simulink model "untitled"  (R2021a)
settings: Solver=VariableStepAuto  StartTime=0.0  StopTime=10  RelTol=1e-3
undefined symbols (not defined in the file or in its folder): magnitude, X, Y, Z
libraries: nesl_utility x14, sm_lib x7, aerolibnav x4, ee_lib x1
settings Model: Creator=thana  LastModifiedBy=thana
settings ExplorerConfigSet: InternalSimMechanicsExplorerSettings="<ExplorerConfiguration><canonicalview>planar_xy</canonicalview><AnimationSetting><BasePlaybackSpeed>1.0</BasePlaybackSpeed><PlaybackSpeedFactor>0.00390625</PlaybackSpeedFactor></AnimationSetting><TilePanel><TileInfo><Tiles Columns=\"1\" Count=\"1\" Rows=\"1\"><Column Weight=\"1\"/><Row Weight=\"1\"/><Tile Height=\"1\" Width=\"1\" X=\"0\" Y=\"0\"/></Tiles></TileInfo><SceneInfo><SceneViewer><BGColor><R>0.60000002384185791</R><G>0.60000002384185791</G><B>0.60000002384185791</B></BGColor><Camera><DoPerspective>off</DoPerspective><Position><X>2.0991662970671161</X><Y>0.871103005730942015</Y><Z>-1.04776641856039454</Z></Position><Center><X>1.45833360517725996</X><Y>0.230270313841087176</Y><Z>-1.68859911045024957</Z></Center><Up><X>-0.408248290463863073</X><Y>0.816496580927726145</Y><Z>-0.408248290463863073</Z></Up><ViewLimDist>1</ViewLimDist><YLim>3.10083582958057757</YLim><XLim>7.0270740022869207</XLim></Camera></SceneViewer></SceneInfo></TilePanel><MechEditorPanel><Cameras/><GfxPanelCameraMap/><VideoCreator><PlaybackSpeedRatio>1.0</PlaybackSpeedRatio><FrameRate>30</FrameRate><VideoFormat>Motion JPEG AVI</VideoFormat><FrameSize>auto</FrameSize></VideoCreator></MechEditorPanel></ExplorerConfiguration>"

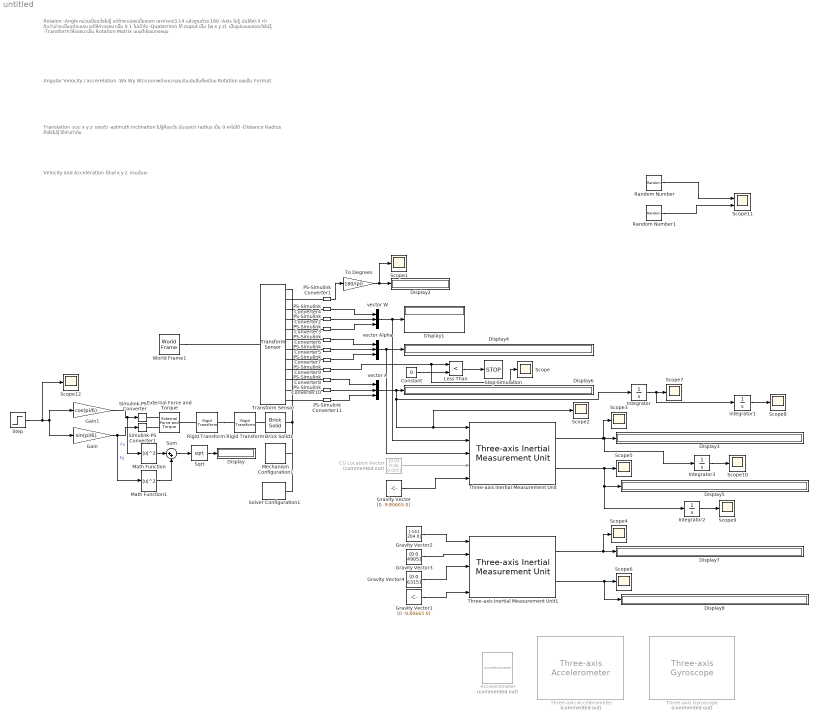
== system untitled ==
  note: Angular Velocity / accerelation
      | -Wx Wy Wz ตามภาพข้างขวาเลย
      |
      | ส่วนอันอื่นก็เหมือน Rotation เลยเป็น Format
  note: Rotaion
      | -Angle หน่วยเป็นอะไรไม่รู้ แต่ถ้าจะแปลงเป็นองศา เอาค่าหาร3.14 แล้วคูณด้วย 180
      | -Axis ไม่รู้ มันให้ค่า 3 ค่า คิดว่าน่าจะเป็นแต่ละแกน แต่ให้ค่าออกมาเป็น 0 1 ไม่เข้าใจ
      | -Quaternion ให้ ouput เป็น [w x y z] เป็นรูปแบบของอะไรไม่รู้
      | -Transform ให้ออกมาเป็น Rotation Matrix แบบที่เรียนจารหยุน
  note: Translation
      | -ระยะ x y z ตรงตัว
      | -azimuth inclination ไม่รู้คืออะไร มันบอกว่า radius เป็น 0 หาไม่ได้
      | -Distance Radius คือไรไม่รู้ ได้ค่าเท่ากัน
  note: Velocity and Acceleration
      | -ได้แค่ x y z ตามนั้นอะ
  Accelerometer : ee_lib/Sensors & Transducers/Accelerometer  Commented=on  output_type=1  sensitivity=1000 mV/gee  sensitivity_pwm=10 1/gee  v_null=2.5 V  duty_cycle0=50  v_max=4 V  duty_cycle_max=75  v_min=1 V  duty_cycle_min=25  F=1000 Hz  Vm=5 V  model_dynamics=0  bw=3 kHz  a_meas_specify=off  a_meas_priority=Low  a_meas=0 m/s^2  a_meas_nominal_specify=off  a_meas_nominal_unit=m/s^2  a_meas_nominal_value=1
      settings: SourceProductBaseCode=PS  InternalSimscapePortConfiguration="{\"Bottom\":[],\"Left\":[{\"id\":\"R\",\"label\":\"R\",\"type\":\"foundation.mechanical.translational.translational\"}],\"Right\":[{\"id\":\"p\",\"label\":\"+\",\"type\":\"foundation.electrical.electrical\"},{\"id\":\"n\",\"label\":\"-\",\"type\":\"foundation.electrical.electrical\"}],\"Top\":[]}"
  Brick Solid1 : sm_lib/Body Elements/Brick Solid  GraphicAmbientColor=[0.15 0.15 0.15 1.0]  BasedOnType=Mass  BrickDimensions=[6 12 1]  BrickDimensionUnits=cm  CenterOfMass=[0 0 0]  CenterOfMassUnits=m  GraphicDiffuseColor=[0.5 0.5 0.5]  Density=2710  DensityUnits=kg/m^3  DoExposeReferenceFrame=on  GraphicEmissiveColor=[0.0 0.0 0.0 1.0]  ExportEntireGeometry=off  SerializedFrames=<Frames><Frame><Id>Frame1</Id><Value><Name>F1</Name><Origin><Source>CenterOfMassFrame</Source><FeatureName></FeatureName></Origin><PrimaryAxis><DefinedDirection>+Z</DefinedDirection><Source>ReferenceFrame</Source><SourceDirection>+Z</SourceDirection><FeatureName></FeatureName></PrimaryAxis><SecondaryAxis><DefinedDirection>+X</DefinedDirection><Source>ReferenceFrame</Source><SourceDirection>+X</SourceDirection><FeatureName></FeatureName></SecondaryAxis></Value></Frame></Frames>  MarkerShape=Sphere  MarkerSize=10  GraphicType=FromGeometry  InertiaType=CalculateFromGeometry  Mass=0.1951  MassUnits=kg  MomentsOfInertia=[1 1 1]  MomentsOfInertiaUnits=kg*m^2  GraphicOpacity=1.0  ProductsOfInertia=[0 0 0]  ProductsOfInertiaUnits=kg*m^2  GraphicShininess=75  GraphicSpecularColor=[0.5 0.5 0.5 1.0]  GraphicVisPropType=SimpleVisualProperties
  CG Location Vector : Constant  Commented=on  Value=[0.03 0.06 0.005]
  Constant : Constant  Value=0
  Display{,1..8} (9 alike) : Display
  External Force and Torque : sm_lib/Forces and Torques/External Force and Torque  ForceResolutionFrame=AttachedFrame  EnableForceX=on  EnableForceY=on  EnableForceZ=off  EnableForce=off  TorqueResolutionFrame=AttachedFrame  EnableTorqueX=off  EnableTorqueY=off  EnableTorqueZ=off  EnableTorque=off
  Gain : Gain  Gain=sin(pi/6)
  Gain1 : Gain  Gain=cos(pi/6)
  Gravity Vector : Constant  Value=[0 -9.80665 0]
  Gravity Vector1 : Constant  Value=[0 -9.80665 0]
  Gravity Vector2 : Constant  Value=[-141 204 0]
  Gravity Vector3 : Constant  Value=[0 0 4905]
  Gravity Vector4 : Constant  Value=[0 0 6315]
  Integrator{,1..3} (4 alike) : Integrator
  Less Than : RelationalOperator  Operator=<  OutDataTypeStr=boolean  RndMeth=Simplest
  Math Function : Math  Operator=magnitude^2  SaturateOnIntegerOverflow=on
  Math Function1 : Math  Operator=magnitude^2  SaturateOnIntegerOverflow=on
  Mechanism Configuration1 : sm_lib/Utilities/Mechanism Configuration  UniformGravity=Constant  GravityVector=[0 -9.80665 0]  GravityVectorUnits=m/s^2  GravityUnits=m/s^2  LinearizationDelta=0.001  JointModeTransitionNonlinearIterations=2
  PS-Simulink Converter{1..11} (11 alike) : nesl_utility/PS-Simulink Converter  PhysicalDomain=network_engine_domain  SubClassName=ps_output  LeftPortType=input  RightPortType=output  PseudoPeriodic=off  Frequencies=[]  Unit=inherit  AffineConversion=off
      settings: SourceProductBaseCode=PW,SS
  Random Number : RandomNumber  SampleTime=0.1
  Random Number1 : RandomNumber  Variance=2  SampleTime=0.1
  Rigid Transform : sm_lib/Frames and Transforms/Rigid Transform  TranslationMethod=Cartesian  TranslationStandardOffset=0  TranslationLengthUnit=cm  TranslationStandardAxis=+Z  TranslationCartesianOffset=[3 6 0]  TranslationROffset=0  TranslationROffsetUnits=m  TranslationZOffset=0  TranslationZOffsetUnits=m  TranslationThetaOffset=0  TranslationThetaOffsetUnits=deg  RotationMethod=None  RotationAngleUnits=deg  RotationStandardAxis=+Z  RotationAngle=0.0  RotationArbitraryAxis=[0 0 1]  FollAlignAxisA=+X  BaseAlignAxisA=+Y  FollAlignAxisB=+Y  BaseAlignAxisB=+Z  RotationSequenceAxes=FollowerAxes  RotationSequence=XYX  RotationSequenceAngles=[0 0 0]  RotationSequenceAnglesUnits=deg  RotationMatrix=[1 0 0; 0 1 0; 0 0 1]
  Rigid Transform1 : sm_lib/Frames and Transforms/Rigid Transform  TranslationMethod=None  TranslationStandardOffset=0  TranslationLengthUnit=cm  TranslationStandardAxis=+Z  TranslationCartesianOffset=[3 6 0]  TranslationROffset=0  TranslationROffsetUnits=m  TranslationZOffset=0  TranslationZOffsetUnits=m  TranslationThetaOffset=0  TranslationThetaOffsetUnits=deg  RotationMethod=None  RotationAngleUnits=deg  RotationStandardAxis=+Z  RotationAngle=0.0  RotationArbitraryAxis=[0 0 1]  FollAlignAxisA=+X  BaseAlignAxisA=+Y  FollAlignAxisB=+Y  BaseAlignAxisB=+Z  RotationSequenceAxes=FollowerAxes  RotationSequence=XYX  RotationSequenceAngles=[0 0 0]  RotationSequenceAnglesUnits=deg  RotationMatrix=[1 0 0; 0 1 0; 0 0 1]
  Scope{,1..10,12} (12 alike) : Scope
  Scope11 : Scope  NumInputPorts=2
  Simulink-PS Converter : nesl_utility/Simulink-PS Converter  PhysicalDomain=network_engine_domain  SubClassName=ps_input  LeftPortType=input  RightPortType=output  PseudoPeriodic=off  Frequencies=[]  NoiseDistribution=none  NoiseParameters=[]  Unit=N  AffineConversion=off  FilteringAndDerivatives=provide  SimscapeFilterOrder=1  InputFilterTimeConstant=0.001  UdotUserProvided=0
      settings: SourceProductBaseCode=PW,SS
  Simulink-PS Converter1 : nesl_utility/Simulink-PS Converter  PhysicalDomain=network_engine_domain  SubClassName=ps_input  LeftPortType=input  RightPortType=output  PseudoPeriodic=off  Frequencies=[]  NoiseDistribution=none  NoiseParameters=[]  Unit=N  AffineConversion=off  FilteringAndDerivatives=provide  SimscapeFilterOrder=1  InputFilterTimeConstant=0.001  UdotUserProvided=0
      settings: SourceProductBaseCode=PW,SS
  Solver Configuration1 : nesl_utility/Solver Configuration  PhysicalDomain=network_engine_domain  SubClassName=solver  LeftPortType=input  RightPortType=generic  Tones=[]  Harmonics=[]  SimulateNoise=off  Profile=off  UseLocalSampling=off  EnableSwitchedLinearOptims=on  FrequencyDomain=off  UseCCode=off  RelTol=0.001  AbsTol=1e-06  MinStep=1e-09  ToWorkspace=off  RevertToSquareIcSolve=off  NumHomotopyIterations=100  PhasorMode=off  PhasorModeNumHarmonics=1  DoDC=off  ResidualTolerance=1e-09  UseLocalSolver=off  LocalSolverChoice=NE_BACKWARD_EULER_ADVANCER  LocalSolverSampleTime=0.001  DoFixedCost=off  MaxNonlinIter=3  MaxModeIter=2  ComputeImpulses=off  ImpulseIterations=2  LinearAlgebra=auto  EquationFormulation=NE_TIME_EF  DelaysMemoryBudget=1024  AutomaticFiltering=on  FilteringTimeConstant=0.001  PartitionStorageMethod=AS_NEEDED  PartitionMemoryBudget=1024  PartitionMethod=ROBUST
      settings: SourceProductBaseCode=PW,SS
  Sqrt : Sqrt  SaturateOnIntegerOverflow=on
  Step : Step  Time=0.01  Before=300  After=0  SampleTime=0
  Stop Simulation : Stop
  Sum : Sum  Inputs=|++
  Three-axis Accelerometer : aerolibnav/Three-axis Accelerometer  Commented=on  units=Metric (MKS)  acc=[0 0 0]  gtype=on  dtype_a=on  w_a=190  z_a=0.707  a_sf_cc=[1 0 0; 0 1 0; 0 0 1]  a_bias=[0 0 0]  a_Ts=0  a_rand=on  a_seeds=[23093 23094 23095]  a_pow=[0.001 0.001 0.001]  a_sat="[-inf  -inf  -inf  inf inf inf]"
      settings: SourceProductBaseCode=AE
  Three-axis Gyroscope : aerolibnav/Three-axis Gyroscope  Commented=on  dtype_g=on  w_g=190  z_g=0.707  g_sf_cc=[1 0 0; 0 1 0; 0 0 1]  g_bias=[0 0 0]  g_sen=[0 0 0]  g_Ts=0  g_rand=on  g_seeds=[23093 23094 23095]  g_pow=[0.0001 0.0001 0.0001]  g_sat="[-inf  -inf  -inf  inf inf inf]"
      settings: SourceProductBaseCode=AE
  Three-axis Inertial Measurement Unit : aerolibnav/Three-axis Inertial Measurement Unit  units=Metric (MKS)  imu=[0 0 0]  i_Ts=0  dtype_a=on  w_a=190  z_a=0.707  a_sf_cc=[1 0 0; 0 1 0; 0 0 1]  a_bias=[0 0 0]  a_sat="[-inf  -inf  -inf  inf inf inf]"  dtype_g=on  w_g=190  z_g=0.707  g_sf_cc=[1 0 0; 0 1 0; 0 0 1]  g_bias=[0 0 0]  g_sens=[0 0 0]  g_sat="[-inf  -inf  -inf  inf inf inf]"  i_rand=on  i_seeds=[23093 23094 23095 23096 23097 23098]  i_pow=[0.001 0.001 0.001 0.0001 0.0001 0.0001]
  Three-axis Inertial Measurement Unit1 : aerolibnav/Three-axis Inertial Measurement Unit  units=Metric (MKS)  imu=[0 0 0]  i_Ts=0  dtype_a=on  w_a=190  z_a=0.707  a_sf_cc=[1 0 0; 0 1 0; 0 0 1]  a_bias=[0 0 0]  a_sat="[-inf  -inf  -inf  inf inf inf]"  dtype_g=on  w_g=190  z_g=0.707  g_sf_cc=[1 0 0; 0 1 0; 0 0 1]  g_bias=[0 0 0]  g_sens=[0 0 0]  g_sat="[-inf  -inf  -inf  inf inf inf]"  i_rand=on  i_seeds=[23093 23094 23095 23096 23097 23098]  i_pow=[0.001 0.001 0.001 0.0001 0.0001 0.0001]
  To Degrees : Gain  Gain=180/(pi)
  Transform Sensor : sm_lib/Frames and Transforms/Transform Sensor  MeasurementFrame=Base  SenseAngle=on  SenseAxis=off  SenseAngle1=off  SenseAngle2=off  SenseAngle3=off  SenseQ=off  SenseR=off  SenseOmegaX=on  SenseOmegaY=on  SenseOmegaZ=on  SenseOmega1=off  SenseOmega2=off  SenseOmega3=off  SenseQDot=off  SenseRDot=off  SenseAlphaX=on  SenseAlphaY=on  SenseAlphaZ=on  SenseAlpha1=off  SenseAlpha2=off  SenseAlpha3=off  SenseQDDot=off  SenseRDDot=off  SenseX=off  SenseY=on  SenseZ=off  SenseRad=off  SenseAzim=off  SenseDist=off  SenseInc=off  SenseXDot=off  SenseYDot=off  SenseZDot=off  SenseRadDot=off  SenseAzimDot=off  SenseDistDot=off  SenseIncDot=off  SenseXDDot=on  SenseYDDot=on  SenseZDDot=on  SenseRadDDot=off  SenseAzimDDot=off  SenseDistDDot=off  SenseIncDDot=off
  World Frame1 : sm_lib/Frames and Transforms/World Frame
  vector A : Concatenate  NumInputs=3
  vector Alpha : Concatenate  NumInputs=3
  vector W : Concatenate  NumInputs=3
  wires:
  Gain1/1 -> Math Function/1, Simulink-PS Converter/1  "Fx"
  Gain/1 -> Simulink-PS Converter1/1, Math Function1/1  "Fy"
  Constant/1 -> Less Than/2
  Less Than/1 -> Stop Simulation/1
  Three-axis Inertial Measurement Unit/1 -> Integrator3/1, Display3/1, Scope3/1
  Three-axis Inertial Measurement Unit/2 -> Integrator2/1, Display5/1, Scope5/1
  vector W/1 -> Display1/1, Three-axis Inertial Measurement Unit/2
  Gravity Vector/1 -> Three-axis Inertial Measurement Unit/5
  CG Location Vector/1 -> Three-axis Inertial Measurement Unit/4
  PS-Simulink Converter1/1 -> To Degrees/1
  To Degrees/1 -> Scope1/1, Display2/1
  PS-Simulink Converter4/1 -> vector W/1
  PS-Simulink Converter2/1 -> vector W/2
  PS-Simulink Converter3/1 -> vector W/3
  PS-Simulink Converter6/1 -> vector Alpha/1
  PS-Simulink Converter5/1 -> vector Alpha/2
  PS-Simulink Converter7/1 -> vector Alpha/3
  vector Alpha/1 -> Display4/1, Three-axis Inertial Measurement Unit/3
  vector A/1 -> Integrator/1, Scope2/1, Three-axis Inertial Measurement Unit/1, Display6/1
  PS-Simulink Converter8/1 -> vector A/1
  PS-Simulink Converter10/1 -> vector A/2
  PS-Simulink Converter11/1 -> vector A/3
  PS-Simulink Converter9/1 -> Scope/1, Less Than/1
  Three-axis Inertial Measurement Unit1/2 -> Scope6/1, Display8/1
  Three-axis Inertial Measurement Unit1/1 -> Display7/1, Scope4/1
  Gravity Vector1/1 -> Three-axis Inertial Measurement Unit1/5
  Gravity Vector2/1 -> Three-axis Inertial Measurement Unit1/1
  Gravity Vector3/1 -> Three-axis Inertial Measurement Unit1/2
  Gravity Vector4/1 -> Three-axis Inertial Measurement Unit1/3
  Integrator/1 -> Integrator1/1, Scope7/1
  Integrator1/1 -> Scope8/1
  Integrator2/1 -> Scope9/1
  Integrator3/1 -> Scope10/1
  Random Number/1 -> Scope11/1
  Random Number1/1 -> Scope11/2
  Math Function/1 -> Sum/1
  Math Function1/1 -> Sum/2
  Sqrt/1 -> Display/1
  Sum/1 -> Sqrt/1
  Step/1 -> Scope12/1, Gain/1, Gain1/1
  connections:
  External Force and Torque/LConn1 -- Simulink-PS Converter/RConn1
  Transform Sensor/RConn1 -- Solver Configuration1/RConn1 -- Mechanism Configuration1/RConn1 -- Brick Solid1/LConn1
  External Force and Torque/LConn2 -- Simulink-PS Converter1/RConn1
  Transform Sensor/RConn3 -- PS-Simulink Converter4/LConn1
  Transform Sensor/RConn2 -- PS-Simulink Converter1/LConn1
  Transform Sensor/RConn4 -- PS-Simulink Converter2/LConn1
  Transform Sensor/RConn5 -- PS-Simulink Converter3/LConn1
  Transform Sensor/RConn6 -- PS-Simulink Converter6/LConn1
  Transform Sensor/RConn7 -- PS-Simulink Converter5/LConn1
  Transform Sensor/RConn8 -- PS-Simulink Converter7/LConn1
  Transform Sensor/RConn9 -- PS-Simulink Converter9/LConn1
  Transform Sensor/RConn10 -- PS-Simulink Converter8/LConn1
  Transform Sensor/RConn11 -- PS-Simulink Converter10/LConn1
  Transform Sensor/RConn12 -- PS-Simulink Converter11/LConn1
  World Frame1/RConn1 -- Transform Sensor/LConn1
  Rigid Transform/RConn1 -- Brick Solid1/RConn1
  Rigid Transform1/LConn1 -- External Force and Torque/RConn1
  Rigid Transform1/RConn1 -- Rigid Transform/LConn1
